simulink model "demo5"  (Simulink 7.1)
settings: Solver=ode45  StartTime=0.0  StopTime=10.0  RelTol=1e-3
libraries: roblocks x7, simulink x1
settings Model: Creator=pic  LastModifiedBy=pic  ExtModeTrigMode=oneshot  ExtModeArmWhenConnect=off
settings DataIOCC: LimitDataPoints=off
settings OptimizationCC: BlockReduction=off  BooleanDataType=off
settings DebuggingCC: SaveWithParameterizedLinksMsg=none  SignalResolutionControl=TryResolveAllWithWarning  SolverPrmCheckMsg=none  MultiTaskDSMMsg=warning  MultiTaskCondExecSysMsg=none  StrictBusMsg=None
settings HardwareCC: TargetUnknown=on
settings RTWCC: IncludeERTFirstTime=on
settings STFCustomTargetCC: ModelReferenceCompliant=off  SystemTargetFile=grt.tlc

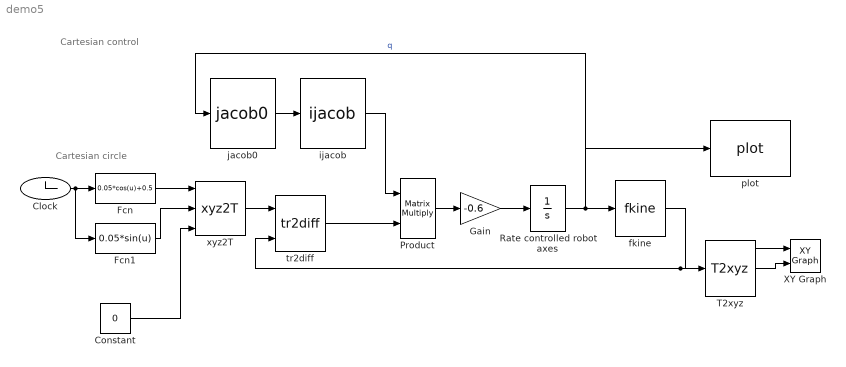
== system demo5 ==
  note: Cartesian circle
  note: Cartesian control
  Clock : Clock
      settings: Decimation=10
  Constant : Constant  Value=0
  Fcn : Fcn  Expr=0.05*cos(u)+0.5
  Fcn1 : Fcn  Expr=0.05*sin(u)
  Gain : Gain  Gain=-0.6  SaturateOnIntegerOverflow=on  OutDataTypeStr=Inherit: Same as input  ParamDataTypeStr=Inherit: Same as input
  Product : Product  Multiplication=Matrix(*)  SaturateOnIntegerOverflow=on  RndMeth=Zero  InputSameDT=on  OutDataTypeStr=Inherit: Same as first input
  Rate controlled robot axes : Integrator  InitialCondition="[0.2763    0.9125    2.9359         0    2.4348   -0.2763]"
  T2xyz : roblocks/T2xyz  SystemSampleTime=-1
  XY Graph : simulink/Sinks/XY Graph  SystemSampleTime=-1  xmin=0.4  xmax=0.6  ymin=-0.1  ymax=0.1  st=-1
  fkine : roblocks/fkine  SystemSampleTime=-1  robot=p560
  ijacob : roblocks/ijacob  SystemSampleTime=-1
  "jacob0 " : roblocks/jacob0   SystemSampleTime=-1  robot=p560
  plot : roblocks/plot  SystemSampleTime=-1  robot=p560
  tr2diff : roblocks/tr2diff  SystemSampleTime=-1  robot=robot
  xyz2T : roblocks/xyz2T  SystemSampleTime=-1
  wires:
  Clock/1 -> Fcn/1, Fcn1/1
  Rate controlled robot axes/1 -> fkine/1, plot/1, "jacob0 "/1  "q"
  Constant/1 -> xyz2T/3
  T2xyz/1 -> XY Graph/1
  T2xyz/2 -> XY Graph/2
  tr2diff/1 -> Product/2
  xyz2T/1 -> tr2diff/1
  fkine/1 -> T2xyz/1, tr2diff/2
  Fcn1/1 -> xyz2T/2
  Fcn/1 -> xyz2T/1
  "jacob0 "/1 -> ijacob/1
  Product/1 -> Gain/1
  ijacob/1 -> Product/1
  Gain/1 -> Rate controlled robot axes/1
